simulink model "KTB1_F"  (R2020a)
settings: Solver=ode45  StartTime=0.0  StopTime=120  RelTol=1e-3
libraries: simulink x8
settings Model: Creator=s182032  LastModifiedBy=morebo
settings DataIOCC: ReturnWorkspaceOutputs=off
settings DebuggingCC: MaxConsecutiveZCsMsg=none  ArithmeticOperatorsInVariantConditions=warning
settings SFSimCC: SimUseLocalCustomCode=off  CustomCodeUndefinedFunction=UseInterfaceOnly
settings RTWCC: RTWUseLocalCustomCode=off

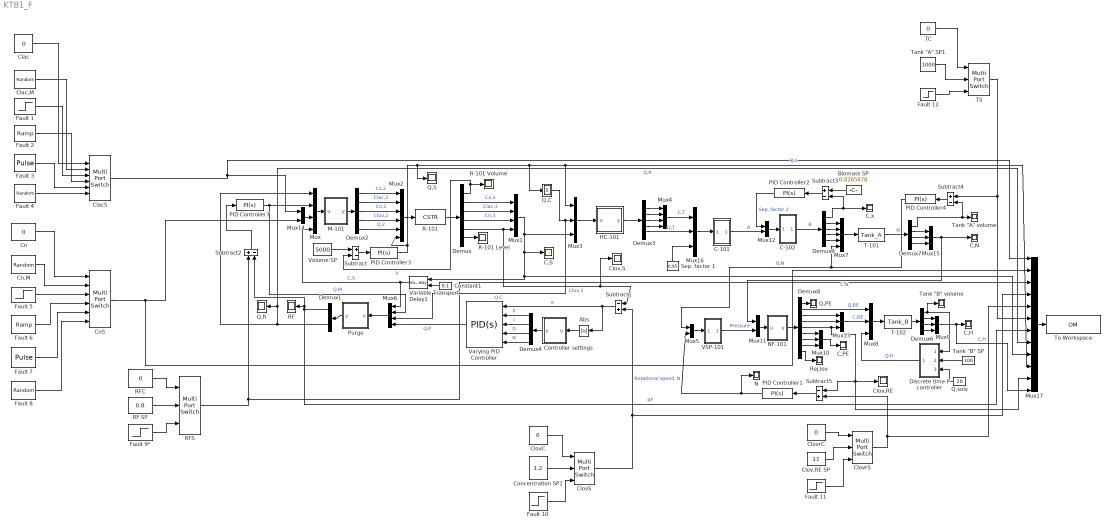
== system KTB1_F ==
  Abs : Abs
  Biomass SP : Constant  Value=0.0265878
  C,H : Scope
  C,N : Scope
  C,PE : Scope
  C,S : Scope
  C,x : Scope
  C-101 : MATLAB Function  TreatAsAtomicUnit=on
  C-102 : MATLAB Function  TreatAsAtomicUnit=on
  Clac : Constant  Value=0
  Clac,M : RandomNumber  Mean=20  Variance=0.001  SampleTime=0.1
  "ClacS " : MultiPortSwitch  DataPortOrder=Zero-based contiguous  Inputs=5  zeroidx=on
  Clov,RE : Scope
  Clov,RE SP : Constant  Value=11
  Clov,S : Scope
  ClovC : Constant  Value=0
  ClovS : MultiPortSwitch  DataPortOrder=Zero-based contiguous  Inputs=2  zeroidx=on
  ClovrC : Constant  Value=0
  "ClovrS " : MultiPortSwitch  DataPortOrder=Zero-based contiguous  Inputs=2  zeroidx=on
  Cn : Constant  Value=0
  Cn,M : RandomNumber  Mean=4  Variance=0.001  SampleTime=0.1
  CnS : MultiPortSwitch  DataPortOrder=Zero-based contiguous  Inputs=5  zeroidx=on
  Concentration SP1 : Constant  Value=1.2
  Constant1 : Constant  Value=0.1
  Controller settings : MATLAB Function  TreatAsAtomicUnit=on
  Demux : Demux  Outputs=6
  Demux1 : Demux  Outputs=2
  Demux2 : Demux  Outputs=5
  Demux3 : Demux  Outputs=5
  Demux4 : Demux
  Demux6 : Demux
  Demux7 : Demux
  Demux8 : Demux  Outputs=9
  Demux9 : Demux  Outputs=5
  Discrete time P controller : Subsystem
  Fault 1 : Step  Time=10  Before=20  After=16  SampleTime=0
  Fault 10 : Step  Time=10.3  Before=1.2  After=1.18  SampleTime=0
  Fault 11 : Step  Before=10.4  After=9  SampleTime=0
  Fault 12 : Step  Time=10.4  Before=1000  After=1050  SampleTime=0
  Fault 2 : simulink/Sources/Ramp  slope=-0.2  start=10  InitialOutput=20
  Fault 3 : DiscretePulseGenerator  Amplitude=20  Period=30  PulseWidth=10  SampleTime=2
  Fault 4 : RandomNumber  Mean=20  Variance=4  SampleTime=0.1
  Fault 5 : Step  Time=10.1  Before=4  After=4.8  SampleTime=0
  Fault 6 : simulink/Sources/Ramp  slope=0.05  start=10  InitialOutput=4
  Fault 7 : DiscretePulseGenerator  Amplitude=4  Period=30  PulseWidth=10  SampleTime=2
  Fault 8 : RandomNumber  Mean=4  Variance=3  SampleTime=0.1
  Fault 9* : Step  Time=10.2  Before=0.8  After=0.84  SampleTime=0
  HC-101 : MATLAB Function  TreatAsAtomicUnit=on
  M-101 : MATLAB Function  TreatAsAtomicUnit=on
  Mux{,1,4,6} (4 alike) : Mux
  Mux{3,8..10,13,15..16} (7 alike) : Mux  Inputs=3
  Mux{5,11..12,14} (4 alike) : Mux  Inputs=2
  Mux17 : Mux  Inputs=12
  Mux2 : Mux  Inputs=6
  Mux7 : Mux  Inputs=5
  N : Scope
  NF-101 : MATLAB Function  TreatAsAtomicUnit=on
  PID Controller1 : simulink/Continuous/PID Controller  Controller=PI  Form=Parallel  TimeDomain=Continuous-time  UseExternalTs=off  SampleTime=-1  IntegratorMethod=Forward Euler  FilterMethod=Forward Euler  ControllerParametersSource=internal  P=0.234567821807165  I=0.999999996666666*0.234567821807165  D=0  UseFilter=on  N=100  TunerSelectOption=Transfer Function Based (PID Tuner App)  InitialConditionSource=internal  InitialConditionForIntegrator=3000  InitialConditionForFilter=0  DifferentiatorICPrevScaledInput=0  ExternalReset=none  TrackingMode=off  Kt=1  LimitOutput=on  UpperSaturationLimit=inf  LowerSaturationLimit=0  LinearizeAsGain=on  AntiWindupMode=clamping  Kb=1  POutMin=[]  POutMax=[]  IOutMin=[]  IOutMax=[]  DOutMin=[]  DOutMax=[]  NOutMin=[]  NOutMax=[]  SumOutMin=[]  SumOutMax=[]  SaturationOutMin=[]  SaturationOutMax=[]  PParamMin=[]  PParamMax=[]  IParamMin=[]  IParamMax=[]  DParamMin=[]  DParamMax=[]  NParamMin=[]  NParamMax=[]  KbParamMin=[]  KbParamMax=[]  KtParamMin=[]  KtParamMax=[]  KbOutMin=[]  KbOutMax=[]  KtOutMin=[]  KtOutMax=[]  IntegratorOutMin=[]  IntegratorOutMax=[]  FilterOutMin=[]  FilterOutMax=[]  SumI1OutMin=[]  SumI1OutMax=[]  SumI2OutMin=[]  SumI2OutMax=[]  SumI3OutMin=[]  SumI3OutMax=[]  SumI4OutMin=[]  SumI4OutMax=[]  SumDOutMin=[]  SumDOutMax=[]  DifferentiatorOutMin=[]  DifferentiatorOutMax=[]  FilterDiffOutCoefMin=[]  FilterDiffOutCoefMax=[]  ReciprocalOutMin=[]  ReciprocalOutMax=[]  SumDenOutMin=[]  SumDenOutMax=[]  SumNumOutMin=[]  SumNumOutMax=[]  DivideOutMin=[]  DivideOutMax=[]  UdiffTsProdOutMin=[]  UdiffTsProdOutMax=[]  NTsProdOutMin=[]  NTsProdOutMax=[]  UintegralTsProdOutMin=[]  UintegralTsProdOutMax=[]  UngainTsProdOutMin=[]  UngainTsProdOutMax=[]  IntegratorContinuousStateAttributes=''  IntegratorStateMustResolveToSignalObject=off  IntegratorRTWStateStorageClass=Auto  FilterContinuousStateAttributes=''  FilterStateMustResolveToSignalObject=off  FilterRTWStateStorageClass=Auto  ParallelPVariant=InternalParameters  IdealPVariant=Disabled  IVariant=InternalParameters  DVariant=Disabled  IntegratorVariant=Continuous  SatVariant=Enabled  AWVariant=ContClampingParallel  PCopyVariant=Disabled  TRVariant=Disabled  FdbkBlocksVariant=Forward  IdealPFdbkVariant=Disabled  SatFdbkVariant=Disabled  DerivativeFilterVariant=Disabled  NVariant=Disabled  NCopyVariant=Disabled_SignalSpec  FilterICVariant=Disabled  IntegratorICVariant=InternalICs  ExternalResetVariant=Disabled  TRSumVariant=Passthrough  SumFdbkVariant=Disabled  SumVariant=Sum_PI  TsampFilterVariant=InternalTs  TsampNgainVariant=Passthrough  TsampIntegralVariant=Passthrough
  PID Controller2 : simulink/Continuous/PID Controller  Controller=PI  Form=Parallel  TimeDomain=Continuous-time  UseExternalTs=off  SampleTime=-1  IntegratorMethod=Forward Euler  FilterMethod=Forward Euler  ControllerParametersSource=internal  P=-0.000476190628986061  I=9.99999996666667*(-0.000476190628986061)  D=0  UseFilter=on  N=100  TunerSelectOption=Transfer Function Based (PID Tuner App)  InitialConditionSource=internal  InitialConditionForIntegrator=0.95  InitialConditionForFilter=0  DifferentiatorICPrevScaledInput=0  ExternalReset=none  TrackingMode=off  Kt=1  LimitOutput=on  UpperSaturationLimit=0.98  LowerSaturationLimit=0  LinearizeAsGain=on  AntiWindupMode=clamping  Kb=1  POutMin=[]  POutMax=[]  IOutMin=[]  IOutMax=[]  DOutMin=[]  DOutMax=[]  NOutMin=[]  NOutMax=[]  SumOutMin=[]  SumOutMax=[]  SaturationOutMin=[]  SaturationOutMax=[]  PParamMin=[]  PParamMax=[]  IParamMin=[]  IParamMax=[]  DParamMin=[]  DParamMax=[]  NParamMin=[]  NParamMax=[]  KbParamMin=[]  KbParamMax=[]  KtParamMin=[]  KtParamMax=[]  KbOutMin=[]  KbOutMax=[]  KtOutMin=[]  KtOutMax=[]  IntegratorOutMin=[]  IntegratorOutMax=[]  FilterOutMin=[]  FilterOutMax=[]  SumI1OutMin=[]  SumI1OutMax=[]  SumI2OutMin=[]  SumI2OutMax=[]  SumI3OutMin=[]  SumI3OutMax=[]  SumI4OutMin=[]  SumI4OutMax=[]  SumDOutMin=[]  SumDOutMax=[]  DifferentiatorOutMin=[]  DifferentiatorOutMax=[]  FilterDiffOutCoefMin=[]  FilterDiffOutCoefMax=[]  ReciprocalOutMin=[]  ReciprocalOutMax=[]  SumDenOutMin=[]  SumDenOutMax=[]  SumNumOutMin=[]  SumNumOutMax=[]  DivideOutMin=[]  DivideOutMax=[]  UdiffTsProdOutMin=[]  UdiffTsProdOutMax=[]  NTsProdOutMin=[]  NTsProdOutMax=[]  UintegralTsProdOutMin=[]  UintegralTsProdOutMax=[]  UngainTsProdOutMin=[]  UngainTsProdOutMax=[]  IntegratorContinuousStateAttributes=''  IntegratorStateMustResolveToSignalObject=off  IntegratorRTWStateStorageClass=Auto  FilterContinuousStateAttributes=''  FilterStateMustResolveToSignalObject=off  FilterRTWStateStorageClass=Auto  ParallelPVariant=InternalParameters  IdealPVariant=Disabled  IVariant=InternalParameters  DVariant=Disabled  IntegratorVariant=Continuous  SatVariant=Enabled  AWVariant=ContClampingParallel  PCopyVariant=Disabled  TRVariant=Disabled  FdbkBlocksVariant=Forward  IdealPFdbkVariant=Disabled  SatFdbkVariant=Disabled  DerivativeFilterVariant=Disabled  NVariant=Disabled  NCopyVariant=Disabled_SignalSpec  FilterICVariant=Disabled  IntegratorICVariant=InternalICs  ExternalResetVariant=Disabled  TRSumVariant=Passthrough  SumFdbkVariant=Disabled  SumVariant=Sum_PI  TsampFilterVariant=InternalTs  TsampNgainVariant=Passthrough  TsampIntegralVariant=Passthrough
  PID Controller3 : simulink/Continuous/PID Controller  Controller=PI  Form=Parallel  TimeDomain=Continuous-time  UseExternalTs=off  SampleTime=-1  IntegratorMethod=Forward Euler  FilterMethod=Forward Euler  ControllerParametersSource=internal  P=-1/0.4/0.2  I=-1/0.4/0.2/4/0.2  D=0  UseFilter=on  N=100  TunerSelectOption=Transfer Function Based (PID Tuner App)  InitialConditionSource=internal  InitialConditionForIntegrator=64.0830509473650  InitialConditionForFilter=0  DifferentiatorICPrevScaledInput=0  ExternalReset=none  TrackingMode=off  Kt=1  LimitOutput=on  UpperSaturationLimit=inf  LowerSaturationLimit=0  LinearizeAsGain=on  AntiWindupMode=clamping  Kb=1  POutMin=[]  POutMax=[]  IOutMin=[]  IOutMax=[]  DOutMin=[]  DOutMax=[]  NOutMin=[]  NOutMax=[]  SumOutMin=[]  SumOutMax=[]  SaturationOutMin=[]  SaturationOutMax=[]  PParamMin=[]  PParamMax=[]  IParamMin=[]  IParamMax=[]  DParamMin=[]  DParamMax=[]  NParamMin=[]  NParamMax=[]  KbParamMin=[]  KbParamMax=[]  KtParamMin=[]  KtParamMax=[]  KbOutMin=[]  KbOutMax=[]  KtOutMin=[]  KtOutMax=[]  IntegratorOutMin=[]  IntegratorOutMax=[]  FilterOutMin=[]  FilterOutMax=[]  SumI1OutMin=[]  SumI1OutMax=[]  SumI2OutMin=[]  SumI2OutMax=[]  SumI3OutMin=[]  SumI3OutMax=[]  SumI4OutMin=[]  SumI4OutMax=[]  SumDOutMin=[]  SumDOutMax=[]  DifferentiatorOutMin=[]  DifferentiatorOutMax=[]  FilterDiffOutCoefMin=[]  FilterDiffOutCoefMax=[]  ReciprocalOutMin=[]  ReciprocalOutMax=[]  SumDenOutMin=[]  SumDenOutMax=[]  SumNumOutMin=[]  SumNumOutMax=[]  DivideOutMin=[]  DivideOutMax=[]  UdiffTsProdOutMin=[]  UdiffTsProdOutMax=[]  NTsProdOutMin=[]  NTsProdOutMax=[]  UintegralTsProdOutMin=[]  UintegralTsProdOutMax=[]  UngainTsProdOutMin=[]  UngainTsProdOutMax=[]  IntegratorContinuousStateAttributes=''  IntegratorStateMustResolveToSignalObject=off  IntegratorRTWStateStorageClass=Auto  FilterContinuousStateAttributes=''  FilterStateMustResolveToSignalObject=off  FilterRTWStateStorageClass=Auto  ParallelPVariant=InternalParameters  IdealPVariant=Disabled  IVariant=InternalParameters  DVariant=Disabled  IntegratorVariant=Continuous  SatVariant=Enabled  AWVariant=ContClampingParallel  PCopyVariant=Disabled  TRVariant=Disabled  FdbkBlocksVariant=Forward  IdealPFdbkVariant=Disabled  SatFdbkVariant=Disabled  DerivativeFilterVariant=Disabled  NVariant=Disabled  NCopyVariant=Disabled_SignalSpec  FilterICVariant=Disabled  IntegratorICVariant=InternalICs  ExternalResetVariant=Disabled  TRSumVariant=Passthrough  SumFdbkVariant=Disabled  SumVariant=Sum_PI  TsampFilterVariant=InternalTs  TsampNgainVariant=Passthrough  TsampIntegralVariant=Passthrough
  PID Controller4 : simulink/Continuous/PID Controller  Controller=PI  Form=Parallel  TimeDomain=Continuous-time  UseExternalTs=off  SampleTime=-1  IntegratorMethod=Forward Euler  FilterMethod=Forward Euler  ControllerParametersSource=internal  P=-1/140  I=-1/4/140/140  D=0  UseFilter=on  N=100  TunerSelectOption=Transfer Function Based (PID Tuner App)  InitialConditionSource=internal  InitialConditionForIntegrator=25.6332203789471  InitialConditionForFilter=0  DifferentiatorICPrevScaledInput=0  ExternalReset=none  TrackingMode=off  Kt=1  LimitOutput=on  UpperSaturationLimit=inf  LowerSaturationLimit=0  LinearizeAsGain=on  AntiWindupMode=clamping  Kb=1  POutMin=[]  POutMax=[]  IOutMin=[]  IOutMax=[]  DOutMin=[]  DOutMax=[]  NOutMin=[]  NOutMax=[]  SumOutMin=[]  SumOutMax=[]  SaturationOutMin=[]  SaturationOutMax=[]  PParamMin=[]  PParamMax=[]  IParamMin=[]  IParamMax=[]  DParamMin=[]  DParamMax=[]  NParamMin=[]  NParamMax=[]  KbParamMin=[]  KbParamMax=[]  KtParamMin=[]  KtParamMax=[]  KbOutMin=[]  KbOutMax=[]  KtOutMin=[]  KtOutMax=[]  IntegratorOutMin=[]  IntegratorOutMax=[]  FilterOutMin=[]  FilterOutMax=[]  SumI1OutMin=[]  SumI1OutMax=[]  SumI2OutMin=[]  SumI2OutMax=[]  SumI3OutMin=[]  SumI3OutMax=[]  SumI4OutMin=[]  SumI4OutMax=[]  SumDOutMin=[]  SumDOutMax=[]  DifferentiatorOutMin=[]  DifferentiatorOutMax=[]  FilterDiffOutCoefMin=[]  FilterDiffOutCoefMax=[]  ReciprocalOutMin=[]  ReciprocalOutMax=[]  SumDenOutMin=[]  SumDenOutMax=[]  SumNumOutMin=[]  SumNumOutMax=[]  DivideOutMin=[]  DivideOutMax=[]  UdiffTsProdOutMin=[]  UdiffTsProdOutMax=[]  NTsProdOutMin=[]  NTsProdOutMax=[]  UintegralTsProdOutMin=[]  UintegralTsProdOutMax=[]  UngainTsProdOutMin=[]  UngainTsProdOutMax=[]  IntegratorContinuousStateAttributes=''  IntegratorStateMustResolveToSignalObject=off  IntegratorRTWStateStorageClass=Auto  FilterContinuousStateAttributes=''  FilterStateMustResolveToSignalObject=off  FilterRTWStateStorageClass=Auto  ParallelPVariant=InternalParameters  IdealPVariant=Disabled  IVariant=InternalParameters  DVariant=Disabled  IntegratorVariant=Continuous  SatVariant=Enabled  AWVariant=ContClampingParallel  PCopyVariant=Disabled  TRVariant=Disabled  FdbkBlocksVariant=Forward  IdealPFdbkVariant=Disabled  SatFdbkVariant=Disabled  DerivativeFilterVariant=Disabled  NVariant=Disabled  NCopyVariant=Disabled_SignalSpec  FilterICVariant=Disabled  IntegratorICVariant=InternalICs  ExternalResetVariant=Disabled  TRSumVariant=Passthrough  SumFdbkVariant=Disabled  SumVariant=Sum_PI  TsampFilterVariant=InternalTs  TsampNgainVariant=Passthrough  TsampIntegralVariant=Passthrough
  PID Controller7 : simulink/Continuous/PID Controller  Controller=PI  Form=Parallel  TimeDomain=Continuous-time  UseExternalTs=off  SampleTime=-1  IntegratorMethod=Forward Euler  FilterMethod=Forward Euler  ControllerParametersSource=internal  P=4.68116891262785/100  I=30.3539293345611/100  D=0  UseFilter=on  N=100  TunerSelectOption=Transfer Function Based (PID Tuner App)  InitialConditionSource=internal  InitialConditionForIntegrator=35.6016949707568  InitialConditionForFilter=0  DifferentiatorICPrevScaledInput=0  ExternalReset=none  TrackingMode=off  Kt=1  LimitOutput=on  UpperSaturationLimit=inf  LowerSaturationLimit=0  LinearizeAsGain=on  AntiWindupMode=clamping  Kb=1  POutMin=[]  POutMax=[]  IOutMin=[]  IOutMax=[]  DOutMin=[]  DOutMax=[]  NOutMin=[]  NOutMax=[]  SumOutMin=[]  SumOutMax=[]  SaturationOutMin=[]  SaturationOutMax=[]  PParamMin=[]  PParamMax=[]  IParamMin=[]  IParamMax=[]  DParamMin=[]  DParamMax=[]  NParamMin=[]  NParamMax=[]  KbParamMin=[]  KbParamMax=[]  KtParamMin=[]  KtParamMax=[]  KbOutMin=[]  KbOutMax=[]  KtOutMin=[]  KtOutMax=[]  IntegratorOutMin=[]  IntegratorOutMax=[]  FilterOutMin=[]  FilterOutMax=[]  SumI1OutMin=[]  SumI1OutMax=[]  SumI2OutMin=[]  SumI2OutMax=[]  SumI3OutMin=[]  SumI3OutMax=[]  SumI4OutMin=[]  SumI4OutMax=[]  SumDOutMin=[]  SumDOutMax=[]  DifferentiatorOutMin=[]  DifferentiatorOutMax=[]  FilterDiffOutCoefMin=[]  FilterDiffOutCoefMax=[]  ReciprocalOutMin=[]  ReciprocalOutMax=[]  SumDenOutMin=[]  SumDenOutMax=[]  SumNumOutMin=[]  SumNumOutMax=[]  DivideOutMin=[]  DivideOutMax=[]  UdiffTsProdOutMin=[]  UdiffTsProdOutMax=[]  NTsProdOutMin=[]  NTsProdOutMax=[]  UintegralTsProdOutMin=[]  UintegralTsProdOutMax=[]  UngainTsProdOutMin=[]  UngainTsProdOutMax=[]  IntegratorContinuousStateAttributes=''  IntegratorStateMustResolveToSignalObject=off  IntegratorRTWStateStorageClass=Auto  FilterContinuousStateAttributes=''  FilterStateMustResolveToSignalObject=off  FilterRTWStateStorageClass=Auto  ParallelPVariant=InternalParameters  IdealPVariant=Disabled  IVariant=InternalParameters  DVariant=Disabled  IntegratorVariant=Continuous  SatVariant=Enabled  AWVariant=ContClampingParallel  PCopyVariant=Disabled  TRVariant=Disabled  FdbkBlocksVariant=Forward  IdealPFdbkVariant=Disabled  SatFdbkVariant=Disabled  DerivativeFilterVariant=Disabled  NVariant=Disabled  NCopyVariant=Disabled_SignalSpec  FilterICVariant=Disabled  IntegratorICVariant=InternalICs  ExternalResetVariant=Disabled  TRSumVariant=Passthrough  SumFdbkVariant=Disabled  SumVariant=Sum_PI  TsampFilterVariant=InternalTs  TsampNgainVariant=Passthrough  TsampIntegralVariant=Passthrough
  Purge : MATLAB Function  TreatAsAtomicUnit=on
  Q,C : Subsystem
  Q,PE : Scope
  Q,R : Scope
  Q,S : Scope
  Q,solv : Constant  Value=20
  R-101 : S-Function  FunctionName=CSTR  SFunctionDeploymentMode=off  EnableBusSupport=off
  R-101 Level : Scope
  R-101 Volume : Scope
  RF : Scope
  RF SP : Constant  Value=0.8
  RFC : Constant  Value=0
  RFS : MultiPortSwitch  DataPortOrder=Zero-based contiguous  Inputs=2  zeroidx=on
  Rej,lov : Scope
  Sep. factor 1 : Constant  Value=0.95
  Subtract{,2..4} (4 alike) : Sum  Inputs=+-
  Subtract1 : Sum  Inputs=-+
  Subtract5 : Sum  Inputs=-+
  T-101 : S-Function  FunctionName=Tank_A  SFunctionDeploymentMode=off  EnableBusSupport=off
  T-102 : S-Function  FunctionName=Tank_B  SFunctionDeploymentMode=off  EnableBusSupport=off
  TC : Constant  Value=0
  "TS " : MultiPortSwitch  DataPortOrder=Zero-based contiguous  Inputs=2  zeroidx=on
  "Tank \"A\" SP1" : Constant  Value=1000
  "Tank \"A\" volume" : Scope
  "Tank \"B\" SP" : Constant  Value=100
  "Tank \"B\" volume" : Scope
  To Workspace : ToWorkspace  VariableName=OM  SaveFormat=Timeseries  SampleTime=-1
  VSP-101 : MATLAB Function  TreatAsAtomicUnit=on
  Variable Transport Delay1 : VariableTransportDelay  VariableDelayType=Variable transport delay  MaximumDelay=10  InitialOutput=[106.351163614666 14.8096563646109 2.51553709810012 1.20000000000003]  MaximumPoints=80000
  Varying PID Controller : simulink/Continuous/PID Controller  Controller=PID  Form=Parallel  TimeDomain=Continuous-time  UseExternalTs=off  SampleTime=-1  IntegratorMethod=Forward Euler  FilterMethod=Forward Euler  ControllerParametersSource=external  P=1  I=1  D=0  UseFilter=on  N=100  TunerSelectOption=Transfer Function Based (PID Tuner App)  InitialConditionSource=internal  InitialConditionForIntegrator=9.96847459181301  InitialConditionForFilter=0  DifferentiatorICPrevScaledInput=0  ExternalReset=none  TrackingMode=off  Kt=1  LimitOutput=on  UpperSaturationLimit=inf  LowerSaturationLimit=0  LinearizeAsGain=on  AntiWindupMode=none  Kb=1  POutMin=[]  POutMax=[]  IOutMin=[]  IOutMax=[]  DOutMin=[]  DOutMax=[]  NOutMin=[]  NOutMax=[]  SumOutMin=[]  SumOutMax=[]  SaturationOutMin=[]  SaturationOutMax=[]  PParamMin=[]  PParamMax=[]  IParamMin=[]  IParamMax=[]  DParamMin=[]  DParamMax=[]  NParamMin=[]  NParamMax=[]  KbParamMin=[]  KbParamMax=[]  KtParamMin=[]  KtParamMax=[]  KbOutMin=[]  KbOutMax=[]  KtOutMin=[]  KtOutMax=[]  IntegratorOutMin=[]  IntegratorOutMax=[]  FilterOutMin=[]  FilterOutMax=[]  SumI1OutMin=[]  SumI1OutMax=[]  SumI2OutMin=[]  SumI2OutMax=[]  SumI3OutMin=[]  SumI3OutMax=[]  SumI4OutMin=[]  SumI4OutMax=[]  SumDOutMin=[]  SumDOutMax=[]  DifferentiatorOutMin=[]  DifferentiatorOutMax=[]  FilterDiffOutCoefMin=[]  FilterDiffOutCoefMax=[]  ReciprocalOutMin=[]  ReciprocalOutMax=[]  SumDenOutMin=[]  SumDenOutMax=[]  SumNumOutMin=[]  SumNumOutMax=[]  DivideOutMin=[]  DivideOutMax=[]  UdiffTsProdOutMin=[]  UdiffTsProdOutMax=[]  NTsProdOutMin=[]  NTsProdOutMax=[]  UintegralTsProdOutMin=[]  UintegralTsProdOutMax=[]  UngainTsProdOutMin=[]  UngainTsProdOutMax=[]  IntegratorContinuousStateAttributes=''  IntegratorStateMustResolveToSignalObject=off  IntegratorRTWStateStorageClass=Auto  FilterContinuousStateAttributes=''  FilterStateMustResolveToSignalObject=off  FilterRTWStateStorageClass=Auto  ParallelPVariant=ExternalParameters  IdealPVariant=Disabled  IVariant=ExternalParameters  DVariant=ExternalParameters  IntegratorVariant=Continuous  SatVariant=Enabled  AWVariant=Passthrough  PCopyVariant=Disabled  TRVariant=Disabled  FdbkBlocksVariant=Forward  IdealPFdbkVariant=Disabled  SatFdbkVariant=Disabled  DerivativeFilterVariant=ContFilter  NVariant=ExternalParameters  NCopyVariant=Disabled  FilterICVariant=InternalICsFilter  IntegratorICVariant=InternalICs  ExternalResetVariant=Disabled  TRSumVariant=Passthrough  SumFdbkVariant=Disabled  SumVariant=Sum_PID  TsampFilterVariant=InternalTs  TsampNgainVariant=Passthrough  TsampIntegralVariant=Passthrough
  Volume SP : Constant  Value=5000
  wires:
  Demux4/1 -> Varying PID Controller/2  "P"
  Subtract1/1 -> Abs/1, Varying PID Controller/1  "e"
  Demux4/2 -> Varying PID Controller/3  "I"
  PID Controller7/1 -> Mux6/2, Mux/2  "Q,M"
  Varying PID Controller/1 -> Mux6/4  "Q,P"
  Demux2/5 -> Mux2/5  "Q,2"
  Mux6/1 -> Purge/1(u)
  Demux2/4 -> Mux2/4  "Clov,2"
  Demux3/1 -> Mux4/1
  Purge/1(y) -> Demux1/1
  Demux2/3 -> Mux2/3  "Cn,2"
  Demux3/2 -> Mux4/2
  Demux3/3 -> Mux4/3
  HC-101/1(y) -> Demux3/1
  Mux3/1 -> HC-101/1(u)
  Demux2/2 -> Mux2/2  "Clac,2"
  PID Controller3/1 -> Mux2/6, Q,S/1, Mux17/10, Mux3/1, Q,C/1(Qs)  "Q,S"
  Demux/1 -> R-101 Volume/1, Subtract/2  "V"
  Demux/2 -> Mux1/1  "Cx,3"
  Demux/3 -> Mux1/2  "Clac,3"
  Mux/1 -> M-101/1(u)
  Mux2/1 -> R-101/1
  Demux2/1 -> Mux2/1  "Cx,2"
  Variable Transport Delay1/1 -> Mux/4, Mux6/1  "C,S"
  R-101/1 -> Demux/1
  Mux1/1 -> C,S/1, Variable Transport Delay1/1, Mux17/9, Mux3/3
  Constant1/1 -> Variable Transport Delay1/2
  M-101/1(y) -> Demux2/1
  Demux/4 -> Mux1/3  "Cn,3"
  Demux/5 -> Clov,S/1, Subtract1/1, Mux1/4  "Clov,3"
  Subtract/1 -> PID Controller3/1
  Demux3/4 -> Mux4/4
  Cn,M/1 -> CnS/2
  Demux/6 -> R-101 Level/1
  Mux14/1 -> Mux/3
  Demux1/2 -> Mux17/8, Q,R/1, Mux/1  "Q,R"
  Volume SP/1 -> Subtract/1
  Demux1/1 -> Mux17/7, RF/1, Subtract2/2  "RF"
  Abs/1 -> Controller settings/1(u)
  Controller settings/1(y) -> Demux4/1
  Demux4/3 -> Varying PID Controller/4  "D"
  Demux4/4 -> Varying PID Controller/5  "N"
  Subtract2/1 -> PID Controller7/1
  Q,C/1(Qc) -> Mux6/3, Mux3/2  "Q,C"
  Demux6/1 -> Discrete time P controller/1(In1), "Tank \"B\" volume"/1
  Discrete time P controller/1(Q,H) -> Mux8/3  "Q,H"
  Q,solv/1 -> Discrete time P controller/3(In3)
  "Tank \"B\" SP"/1 -> Discrete time P controller/2(In2)
  Demux9/4 -> Mux7/3
  Subtract3/1 -> PID Controller2/1
  C-102/1(y) -> Demux9/1  "B"
  Demux8/9 -> Rej,lov/1
  PID Controller1/1 -> Mux5/2, N/1  "Rotational speed, N"
  Demux9/1 -> C,x/1, Subtract3/2
  Demux7/3 -> Mux15/2
  Demux8/8 -> Mux10/3
  Demux9/2 -> Mux7/1
  Mux5/1 -> VSP-101/1(u)
  VSP-101/1(y) -> Mux11/2  "Pressure"
  Demux6/2 -> Mux9/1
  T-102/1 -> Demux6/1
  Demux9/5 -> Mux7/4
  Demux8/2 -> Mux8/1  "Q,RE"
  Demux6/3 -> Mux9/2
  Mux15/1 -> C,N/1, Mux11/1  "C,N"
  Mux7/1 -> T-101/1
  Demux9/3 -> Mux7/2
  Demux8/3 -> Mux13/1
  Demux8/5 -> Mux17/11, Subtract5/1, Clov,RE/1, Mux13/3
  Mux8/1 -> T-102/1
  Mux10/1 -> C,PE/1
  Demux8/4 -> Mux13/2
  Subtract4/1 -> PID Controller4/1
  PID Controller4/1 -> Mux5/1, Mux7/5  "Q,N"
  Subtract5/1 -> PID Controller1/1
  Demux8/7 -> Mux10/2
  Demux6/4 -> Mux9/3
  Demux7/1 -> "Tank \"A\" volume"/1, Subtract4/2
  Mux16/1 -> C-101/1(u)
  Sep. factor 1/1 -> Mux16/3
  Mux11/1 -> NF-101/1(u)
  NF-101/1(y) -> Demux8/1
  Mux9/1 -> Mux17/12, C,H/1  "C,H"
  T-101/1 -> Demux7/1  "N"
  Mux13/1 -> Mux8/2  "C,RE"
  Mux12/1 -> C-102/1(u)
  Biomass SP/1 -> Subtract3/1
  Demux8/6 -> Mux10/1
  Demux7/4 -> Mux15/3
  Demux8/1 -> Q,PE/1
  C-101/1(y) -> Mux12/2  "A"
  Demux7/2 -> Mux15/1
  PID Controller2/1 -> Mux12/1  "Sep. factor 2"
  Mux4/1 -> Mux16/1  "C,T"
  Demux3/5 -> Mux16/2  "Q,T"
  Mux17/1 -> To Workspace/1
  Fault 1/1 -> "ClacS "/3
  Fault 2/1 -> "ClacS "/4
  "ClacS "/1 -> Mux17/1, Mux14/1
  Clac,M/1 -> "ClacS "/2
  Fault 3/1 -> "ClacS "/5
  Fault 4/1 -> "ClacS "/6
  CnS/1 -> Mux17/2, Mux14/2
  Fault 5/1 -> CnS/3
  Fault 6/1 -> CnS/4
  Fault 7/1 -> CnS/5
  Clac/1 -> "ClacS "/1
  Cn/1 -> CnS/1
  Fault 8/1 -> CnS/6
  RFC/1 -> RFS/1
  RF SP/1 -> RFS/2
  Fault 9*/1 -> RFS/3
  RFS/1 -> Subtract2/1, Mux17/3
  ClovrC/1 -> "ClovrS "/1
  "ClovrS "/1 -> Mux17/5, Subtract5/2
  Clov,RE SP/1 -> "ClovrS "/2
  Fault 11/1 -> "ClovrS "/3
  "Tank \"A\" SP1"/1 -> "TS "/2
  TC/1 -> "TS "/1
  Fault 12/1 -> "TS "/3
  "TS "/1 -> Mux17/6, Subtract4/1
  Concentration SP1/1 -> ClovS/2
  ClovC/1 -> ClovS/1
  Fault 10/1 -> ClovS/3
  ClovS/1 -> Mux17/4, Subtract1/2

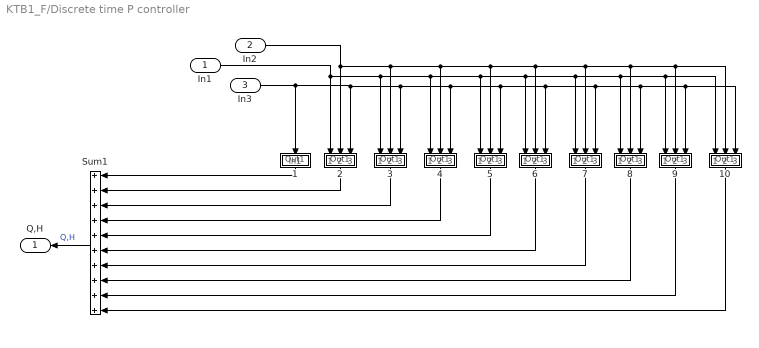
== system KTB1_F/Discrete time P controller ==
  In1 : Inport
  In2 : Inport  Port=2
  In3 : Inport  Port=3
  1 : Subsystem
  10 : Subsystem
  2 : Subsystem
  3 : Subsystem
  4 : Subsystem
  5 : Subsystem
  6 : Subsystem
  7 : Subsystem
  8 : Subsystem
  9 : Subsystem
  Sum1 : Sum  Inputs=++++++++++
  Q,H : Outport  VectorParamsAs1DForOutWhenUnconnected=off
  wires:
  In3/1 -> 3/3(In3), 4/3(In3), 6/3(In3), 7/3(In3), 8/3(In3), 10/3(In3), 9/3(In3), 5/3(In3), 2/3(In3), 1/1(In1)
  In2/1 -> 2/2(In2), 3/2(In2), 4/2(In2), 5/2(In2), 6/2(In2), 8/2(In2), 10/2(In2), 9/2(In2), 7/2(In2)
  7/1(Out1) -> Sum1/7
  3/1(Out1) -> Sum1/3
  4/1(Out1) -> Sum1/4
  2/1(Out1) -> Sum1/2
  6/1(Out1) -> Sum1/6
  8/1(Out1) -> Sum1/8
  10/1(Out1) -> Sum1/10
  9/1(Out1) -> Sum1/9
  5/1(Out1) -> Sum1/5
  Sum1/1 -> Q,H/1  "Q,H"
  1/1(Out1) -> Sum1/1
  In1/1 -> 4/1(In1), 5/1(In1), 6/1(In1), 7/1(In1), 8/1(In1), 10/1(In1), 9/1(In1), 3/1(In1), 2/1(In1)

== system KTB1_F/Q,C ==
  Qs : Inport
  Product1 : Product
  Q,C/Q,S : Constant  Value=0.6
  Qc : Outport  VectorParamsAs1DForOutWhenUnconnected=off
  wires:
  Product1/1 -> Qc/1  "Qc"
  Q,C/Q,S/1 -> Product1/1
  Qs/1 -> Product1/2

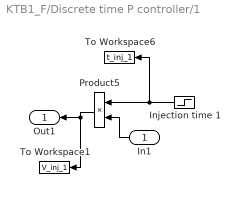
== system KTB1_F/Discrete time P controller/1 ==
  In1 : Inport
  Injection time 1 : Step  Time=(5.1313509526065/20)*6  Before=1  After=0  SampleTime=0
  Product5 : Product
  To Workspace1 : ToWorkspace  VariableName=V_inj_1  SaveFormat=Timeseries  SampleTime=-1
  To Workspace6 : ToWorkspace  VariableName=t_inj_1  SaveFormat=Timeseries  SampleTime=-1
  Out1 : Outport  VectorParamsAs1DForOutWhenUnconnected=off
  wires:
  Product5/1 -> To Workspace1/1, Out1/1
  Injection time 1/1 -> Product5/1, To Workspace6/1
  In1/1 -> Product5/2

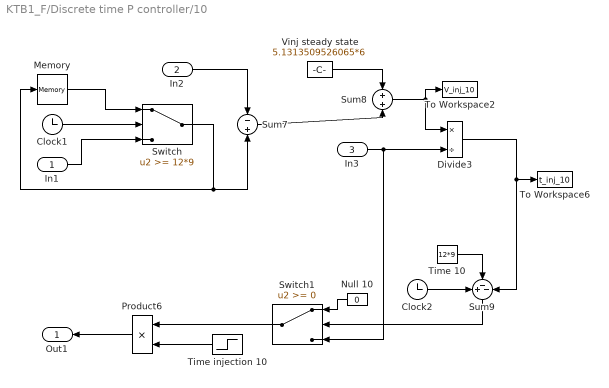
== system KTB1_F/Discrete time P controller/10 ==
  In1 : Inport
  In2 : Inport  Port=2
  In3 : Inport  Port=3
  Clock1 : Clock
  Clock2 : Clock
  Divide3 : Product  Inputs=*/
  Memory : Memory
  Null 10 : Constant  Value=0
  Product6 : Product
  Sum7 : Sum  Inputs=-+
  Sum8 : Sum
  Sum9 : Sum  Inputs=+--
  Switch : Switch  Threshold=12*9
  Switch1 : Switch
  Time 10 : Constant  Value=12*9
  Time injection 10 : Step  Time=12*9  SampleTime=0
  To Workspace2 : ToWorkspace  VariableName=V_inj_10  SaveFormat=Timeseries  SampleTime=-1
  To Workspace6 : ToWorkspace  VariableName=t_inj_10  SaveFormat=Timeseries  SampleTime=-1
  Vinj steady state : Constant  Value=5.1313509526065*6
  Out1 : Outport  VectorParamsAs1DForOutWhenUnconnected=off
  wires:
  In1/1 -> Switch/3
  Time injection 10/1 -> Product6/2
  Switch/1 -> Memory/1, Sum7/2
  Time 10/1 -> Sum9/2
  Switch1/1 -> Product6/1
  Clock1/1 -> Switch/2
  Memory/1 -> Switch/1
  Null 10/1 -> Switch1/1
  Divide3/1 -> Sum9/3, To Workspace6/1
  Clock2/1 -> Sum9/1
  In2/1 -> Sum7/1
  Vinj steady state/1 -> Sum8/1
  In3/1 -> Switch1/3, Divide3/2
  Sum9/1 -> Switch1/2
  Sum7/1 -> Sum8/2
  Product6/1 -> Out1/1
  Sum8/1 -> Divide3/1, To Workspace2/1

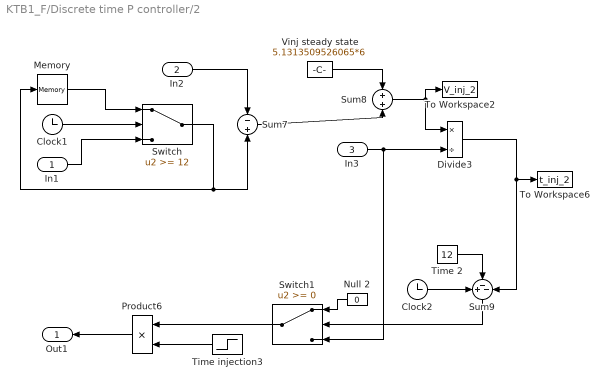
== system KTB1_F/Discrete time P controller/2 ==
  In1 : Inport
  In2 : Inport  Port=2
  In3 : Inport  Port=3
  Clock1 : Clock
  Clock2 : Clock
  Divide3 : Product  Inputs=*/
  Memory : Memory
  Null 2 : Constant  Value=0
  Product6 : Product
  Sum7 : Sum  Inputs=-+
  Sum8 : Sum
  Sum9 : Sum  Inputs=+--
  Switch : Switch  Threshold=12
  Switch1 : Switch
  Time 2 : Constant  Value=12
  Time injection3 : Step  Time=12  SampleTime=0
  To Workspace2 : ToWorkspace  VariableName=V_inj_2  SaveFormat=Timeseries  SampleTime=-1
  To Workspace6 : ToWorkspace  VariableName=t_inj_2  SaveFormat=Timeseries  SampleTime=-1
  Vinj steady state : Constant  Value=5.1313509526065*6
  Out1 : Outport  VectorParamsAs1DForOutWhenUnconnected=off
  wires:
  In1/1 -> Switch/3
  Time injection3/1 -> Product6/2
  Switch/1 -> Memory/1, Sum7/2
  Time 2/1 -> Sum9/2
  Switch1/1 -> Product6/1
  Clock1/1 -> Switch/2
  Memory/1 -> Switch/1
  Null 2/1 -> Switch1/1
  Divide3/1 -> Sum9/3, To Workspace6/1
  Clock2/1 -> Sum9/1
  In2/1 -> Sum7/1
  Vinj steady state/1 -> Sum8/1
  In3/1 -> Switch1/3, Divide3/2
  Sum9/1 -> Switch1/2
  Sum7/1 -> Sum8/2
  Product6/1 -> Out1/1
  Sum8/1 -> Divide3/1, To Workspace2/1

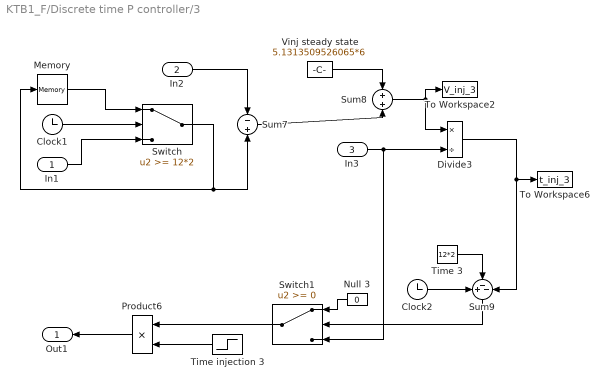
== system KTB1_F/Discrete time P controller/3 ==
  In1 : Inport
  In2 : Inport  Port=2
  In3 : Inport  Port=3
  Clock1 : Clock
  Clock2 : Clock
  Divide3 : Product  Inputs=*/
  Memory : Memory
  Null 3 : Constant  Value=0
  Product6 : Product
  Sum7 : Sum  Inputs=-+
  Sum8 : Sum
  Sum9 : Sum  Inputs=+--
  Switch : Switch  Threshold=12*2
  Switch1 : Switch
  Time 3 : Constant  Value=12*2
  Time injection 3 : Step  Time=12*2  SampleTime=0
  To Workspace2 : ToWorkspace  VariableName=V_inj_3  SaveFormat=Timeseries  SampleTime=-1
  To Workspace6 : ToWorkspace  VariableName=t_inj_3  SaveFormat=Timeseries  SampleTime=-1
  Vinj steady state : Constant  Value=5.1313509526065*6
  Out1 : Outport  VectorParamsAs1DForOutWhenUnconnected=off
  wires:
  In1/1 -> Switch/3
  Time injection 3/1 -> Product6/2
  Switch/1 -> Memory/1, Sum7/2
  Time 3/1 -> Sum9/2
  Switch1/1 -> Product6/1
  Clock1/1 -> Switch/2
  Memory/1 -> Switch/1
  Null 3/1 -> Switch1/1
  Divide3/1 -> Sum9/3, To Workspace6/1
  Clock2/1 -> Sum9/1
  In2/1 -> Sum7/1
  Vinj steady state/1 -> Sum8/1
  In3/1 -> Switch1/3, Divide3/2
  Sum9/1 -> Switch1/2
  Sum7/1 -> Sum8/2
  Product6/1 -> Out1/1
  Sum8/1 -> Divide3/1, To Workspace2/1

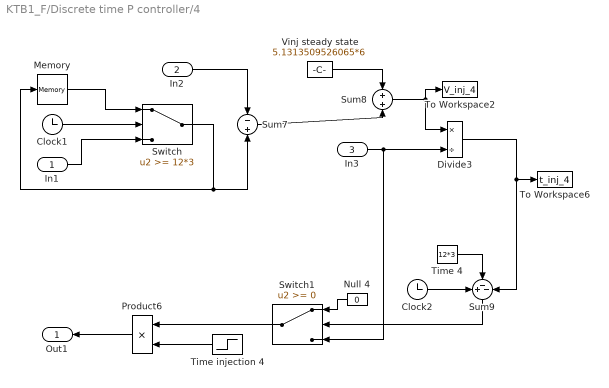
== system KTB1_F/Discrete time P controller/4 ==
  In1 : Inport
  In2 : Inport  Port=2
  In3 : Inport  Port=3
  Clock1 : Clock
  Clock2 : Clock
  Divide3 : Product  Inputs=*/
  Memory : Memory
  Null 4 : Constant  Value=0
  Product6 : Product
  Sum7 : Sum  Inputs=-+
  Sum8 : Sum
  Sum9 : Sum  Inputs=+--
  Switch : Switch  Threshold=12*3
  Switch1 : Switch
  Time 4 : Constant  Value=12*3
  Time injection 4 : Step  Time=12*3  SampleTime=0
  To Workspace2 : ToWorkspace  VariableName=V_inj_4  SaveFormat=Timeseries  SampleTime=-1
  To Workspace6 : ToWorkspace  VariableName=t_inj_4  SaveFormat=Timeseries  SampleTime=-1
  Vinj steady state : Constant  Value=5.1313509526065*6
  Out1 : Outport  VectorParamsAs1DForOutWhenUnconnected=off
  wires:
  In1/1 -> Switch/3
  Time injection 4/1 -> Product6/2
  Switch/1 -> Memory/1, Sum7/2
  Time 4/1 -> Sum9/2
  Switch1/1 -> Product6/1
  Clock1/1 -> Switch/2
  Memory/1 -> Switch/1
  Null 4/1 -> Switch1/1
  Divide3/1 -> Sum9/3, To Workspace6/1
  Clock2/1 -> Sum9/1
  In2/1 -> Sum7/1
  Vinj steady state/1 -> Sum8/1
  In3/1 -> Switch1/3, Divide3/2
  Sum9/1 -> Switch1/2
  Sum7/1 -> Sum8/2
  Product6/1 -> Out1/1
  Sum8/1 -> Divide3/1, To Workspace2/1

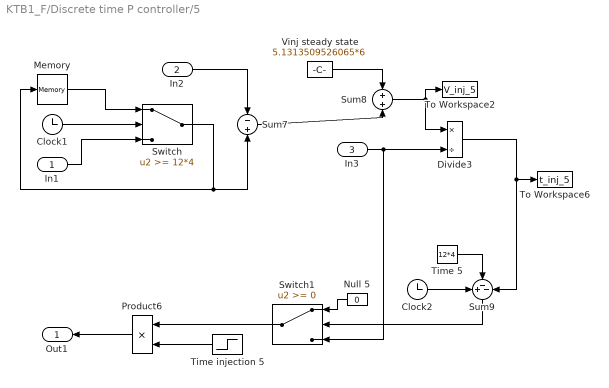
== system KTB1_F/Discrete time P controller/5 ==
  In1 : Inport
  In2 : Inport  Port=2
  In3 : Inport  Port=3
  Clock1 : Clock
  Clock2 : Clock
  Divide3 : Product  Inputs=*/
  Memory : Memory
  Null 5 : Constant  Value=0
  Product6 : Product
  Sum7 : Sum  Inputs=-+
  Sum8 : Sum
  Sum9 : Sum  Inputs=+--
  Switch : Switch  Threshold=12*4
  Switch1 : Switch
  Time 5 : Constant  Value=12*4
  Time injection 5 : Step  Time=12*4  SampleTime=0
  To Workspace2 : ToWorkspace  VariableName=V_inj_5  SaveFormat=Timeseries  SampleTime=-1
  To Workspace6 : ToWorkspace  VariableName=t_inj_5  SaveFormat=Timeseries  SampleTime=-1
  Vinj steady state : Constant  Value=5.1313509526065*6
  Out1 : Outport  VectorParamsAs1DForOutWhenUnconnected=off
  wires:
  In1/1 -> Switch/3
  Time injection 5/1 -> Product6/2
  Switch/1 -> Memory/1, Sum7/2
  Time 5/1 -> Sum9/2
  Switch1/1 -> Product6/1
  Clock1/1 -> Switch/2
  Memory/1 -> Switch/1
  Null 5/1 -> Switch1/1
  Divide3/1 -> Sum9/3, To Workspace6/1
  Clock2/1 -> Sum9/1
  In2/1 -> Sum7/1
  Vinj steady state/1 -> Sum8/1
  In3/1 -> Switch1/3, Divide3/2
  Sum9/1 -> Switch1/2
  Sum7/1 -> Sum8/2
  Product6/1 -> Out1/1
  Sum8/1 -> Divide3/1, To Workspace2/1

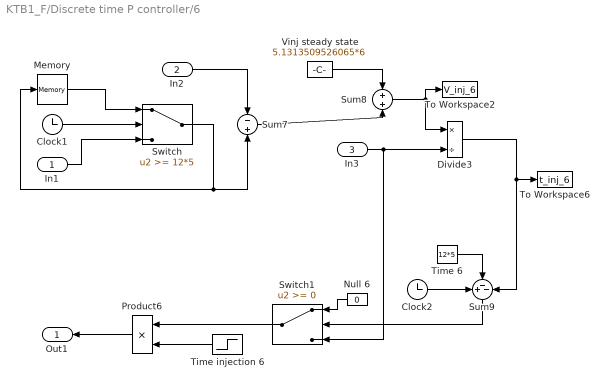
== system KTB1_F/Discrete time P controller/6 ==
  In1 : Inport
  In2 : Inport  Port=2
  In3 : Inport  Port=3
  Clock1 : Clock
  Clock2 : Clock
  Divide3 : Product  Inputs=*/
  Memory : Memory
  Null 6 : Constant  Value=0
  Product6 : Product
  Sum7 : Sum  Inputs=-+
  Sum8 : Sum
  Sum9 : Sum  Inputs=+--
  Switch : Switch  Threshold=12*5
  Switch1 : Switch
  Time 6 : Constant  Value=12*5
  Time injection 6 : Step  Time=12*5  SampleTime=0
  To Workspace2 : ToWorkspace  VariableName=V_inj_6  SaveFormat=Timeseries  SampleTime=-1
  To Workspace6 : ToWorkspace  VariableName=t_inj_6  SaveFormat=Timeseries  SampleTime=-1
  Vinj steady state : Constant  Value=5.1313509526065*6
  Out1 : Outport  VectorParamsAs1DForOutWhenUnconnected=off
  wires:
  In1/1 -> Switch/3
  Time injection 6/1 -> Product6/2
  Switch/1 -> Memory/1, Sum7/2
  Time 6/1 -> Sum9/2
  Switch1/1 -> Product6/1
  Clock1/1 -> Switch/2
  Memory/1 -> Switch/1
  Null 6/1 -> Switch1/1
  Divide3/1 -> Sum9/3, To Workspace6/1
  Clock2/1 -> Sum9/1
  In2/1 -> Sum7/1
  Vinj steady state/1 -> Sum8/1
  In3/1 -> Switch1/3, Divide3/2
  Sum9/1 -> Switch1/2
  Sum7/1 -> Sum8/2
  Product6/1 -> Out1/1
  Sum8/1 -> Divide3/1, To Workspace2/1

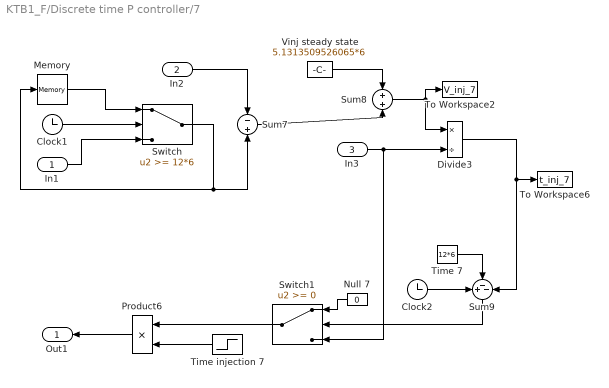
== system KTB1_F/Discrete time P controller/7 ==
  In1 : Inport
  In2 : Inport  Port=2
  In3 : Inport  Port=3
  Clock1 : Clock
  Clock2 : Clock
  Divide3 : Product  Inputs=*/
  Memory : Memory
  Null 7 : Constant  Value=0
  Product6 : Product
  Sum7 : Sum  Inputs=-+
  Sum8 : Sum
  Sum9 : Sum  Inputs=+--
  Switch : Switch  Threshold=12*6
  Switch1 : Switch
  Time 7 : Constant  Value=12*6
  Time injection 7 : Step  Time=12*6  SampleTime=0
  To Workspace2 : ToWorkspace  VariableName=V_inj_7  SaveFormat=Timeseries  SampleTime=-1
  To Workspace6 : ToWorkspace  VariableName=t_inj_7  SaveFormat=Timeseries  SampleTime=-1
  Vinj steady state : Constant  Value=5.1313509526065*6
  Out1 : Outport  VectorParamsAs1DForOutWhenUnconnected=off
  wires:
  In1/1 -> Switch/3
  Time injection 7/1 -> Product6/2
  Switch/1 -> Memory/1, Sum7/2
  Time 7/1 -> Sum9/2
  Switch1/1 -> Product6/1
  Clock1/1 -> Switch/2
  Memory/1 -> Switch/1
  Null 7/1 -> Switch1/1
  Divide3/1 -> Sum9/3, To Workspace6/1
  Clock2/1 -> Sum9/1
  In2/1 -> Sum7/1
  Vinj steady state/1 -> Sum8/1
  In3/1 -> Switch1/3, Divide3/2
  Sum9/1 -> Switch1/2
  Sum7/1 -> Sum8/2
  Product6/1 -> Out1/1
  Sum8/1 -> Divide3/1, To Workspace2/1

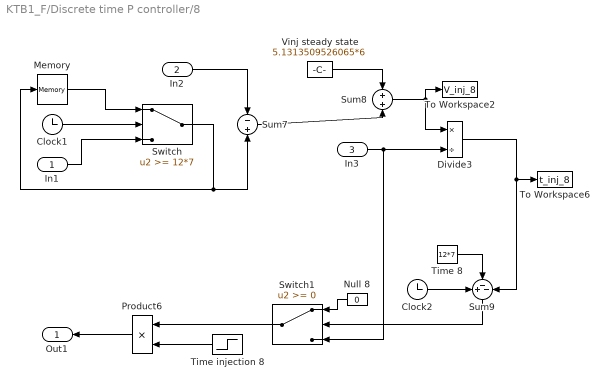
== system KTB1_F/Discrete time P controller/8 ==
  In1 : Inport
  In2 : Inport  Port=2
  In3 : Inport  Port=3
  Clock1 : Clock
  Clock2 : Clock
  Divide3 : Product  Inputs=*/
  Memory : Memory
  Null 8 : Constant  Value=0
  Product6 : Product
  Sum7 : Sum  Inputs=-+
  Sum8 : Sum
  Sum9 : Sum  Inputs=+--
  Switch : Switch  Threshold=12*7
  Switch1 : Switch
  Time 8 : Constant  Value=12*7
  Time injection 8 : Step  Time=12*7  SampleTime=0
  To Workspace2 : ToWorkspace  VariableName=V_inj_8  SaveFormat=Timeseries  SampleTime=-1
  To Workspace6 : ToWorkspace  VariableName=t_inj_8  SaveFormat=Timeseries  SampleTime=-1
  Vinj steady state : Constant  Value=5.1313509526065*6
  Out1 : Outport  VectorParamsAs1DForOutWhenUnconnected=off
  wires:
  In1/1 -> Switch/3
  Time injection 8/1 -> Product6/2
  Switch/1 -> Memory/1, Sum7/2
  Time 8/1 -> Sum9/2
  Switch1/1 -> Product6/1
  Clock1/1 -> Switch/2
  Memory/1 -> Switch/1
  Null 8/1 -> Switch1/1
  Divide3/1 -> Sum9/3, To Workspace6/1
  Clock2/1 -> Sum9/1
  In2/1 -> Sum7/1
  Vinj steady state/1 -> Sum8/1
  In3/1 -> Switch1/3, Divide3/2
  Sum9/1 -> Switch1/2
  Sum7/1 -> Sum8/2
  Product6/1 -> Out1/1
  Sum8/1 -> Divide3/1, To Workspace2/1

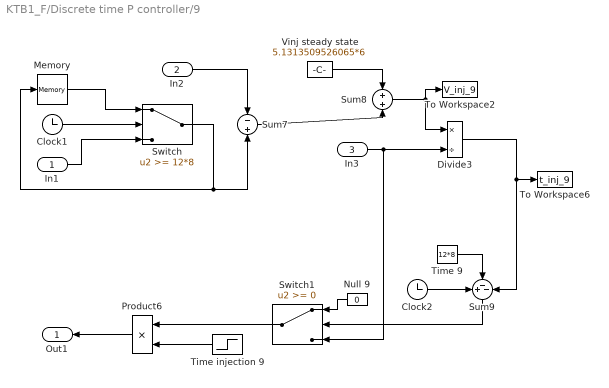
== system KTB1_F/Discrete time P controller/9 ==
  In1 : Inport
  In2 : Inport  Port=2
  In3 : Inport  Port=3
  Clock1 : Clock
  Clock2 : Clock
  Divide3 : Product  Inputs=*/
  Memory : Memory
  Null 9 : Constant  Value=0
  Product6 : Product
  Sum7 : Sum  Inputs=-+
  Sum8 : Sum
  Sum9 : Sum  Inputs=+--
  Switch : Switch  Threshold=12*8
  Switch1 : Switch
  Time 9 : Constant  Value=12*8
  Time injection 9 : Step  Time=12*8  SampleTime=0
  To Workspace2 : ToWorkspace  VariableName=V_inj_9  SaveFormat=Timeseries  SampleTime=-1
  To Workspace6 : ToWorkspace  VariableName=t_inj_9  SaveFormat=Timeseries  SampleTime=-1
  Vinj steady state : Constant  Value=5.1313509526065*6
  Out1 : Outport  VectorParamsAs1DForOutWhenUnconnected=off
  wires:
  In1/1 -> Switch/3
  Time injection 9/1 -> Product6/2
  Switch/1 -> Memory/1, Sum7/2
  Time 9/1 -> Sum9/2
  Switch1/1 -> Product6/1
  Clock1/1 -> Switch/2
  Memory/1 -> Switch/1
  Null 9/1 -> Switch1/1
  Divide3/1 -> Sum9/3, To Workspace6/1
  Clock2/1 -> Sum9/1
  In2/1 -> Sum7/1
  Vinj steady state/1 -> Sum8/1
  In3/1 -> Switch1/3, Divide3/2
  Sum9/1 -> Switch1/2
  Sum7/1 -> Sum8/2
  Product6/1 -> Out1/1
  Sum8/1 -> Divide3/1, To Workspace2/1

== matlab function KTB1_F/M-101 ==
  data: y output; u input
function y  = MX(u) 

% inputs
Q_R = u(1);
Q_M = u(2);
C_LAC_M = u(3);
C_N_M = u(4);
C_X_S = u(5);
C_LAC_S = u(6);
C_N_S = u(7);
C_MEV_S = u(8);

%C_LAC_M=10;
%C_N_M=2;

beta=1.9;

%remember C_LAC_R=C_LAC_S C_N_R=C_N_S

y=zeros(5,1);
y(1) = C_X_S*beta*Q_R/(Q_M+Q_R); %C_X_F
y(2) = (C_LAC_M*Q_M+C_LAC_S*Q_R)/(Q_M+Q_R); %C_LAC_F
y(3) = (C_N_M*Q_M+C_N_S*Q_R)/(Q_M+Q_R); %C_N_F
y(4) = C_MEV_S*Q_R/(Q_M+Q_R); %C_MEV_F
y(5) = (Q_M+Q_R); % Q_F

== matlab function KTB1_F/C-101 ==
  data: u input size=6; y output
 function y  = CF1(u)
% X=0.99; %separation factor
%Q4=QP1; volumetric capacity of the centrifuge

%inputs
C_X_T = u(1);
C_LAC_T = u(2);
C_N_T = u(3);
C_MEV_T = u(4);
Q_T = u(5);
X = u(6);

y=zeros(5,1);

y(1)=(1-X)*C_X_T;
y(2)=C_LAC_T;
y(3)=C_N_T;
y(4)=C_MEV_T;
y(5)= Q_T;

== matlab function KTB1_F/Purge ==
  data: u input size=7; y output
function y = PU(u)

% inputs
C_X_S = u(1);
C_LAC_S = u(2);
C_N_S = u(3);
C_MEV_S = u(4);
Q_M=u(5);
Q_C=u(6);
Q_P=u(7);

%F_purge=0.13;
%R=0.8;
% Q1=1.6; %l/h
%QC=1.8;
% F_purge*Q_C
%Q_P=Q_C-0.8*Q_1;

y=zeros(2,1);
y(1) = (Q_C-Q_P)/Q_M; % RR
y(2) = (Q_C-Q_P); % Q_R

== matlab function KTB1_F/C-102 ==
  data: u input size=6; y output
 function y  = CF2(u)
% X=0.99; %separation factor
%Q4=QP1; volumetric capacity of the centrifuge

%inputs
X = u(1); %separation factor
C_X_T = u(2);
C_LAC_T = u(3);
C_N_T = u(4);
C_MEV_T = u(5);
Q_T = u(6);


y=zeros(5,1);

y(1)=(1-X)*C_X_T;
y(2)=C_LAC_T;
y(3)=C_N_T;
y(4)=C_MEV_T;
y(5)= Q_T;

== matlab function KTB1_F/VSP-101 ==
  data: u input size=2; y output size=2
function y  = VSP(u)

%input
%time=u(1);
Q=u(1);
n=u(2);

dim=2;

y=zeros(dim,1);

% output

y(1)=Q;
y(2)=(-0.085*Q^2 - 0.0000329*Q*n + 0.0000155555555555556*n^2)/10.2024665317458;

% -0.085x^(2)-0.0000329*2900x+0.0000155555555555556*2900

%10.199773339984

end

== matlab function KTB1_F/NF-101 ==
  data: u input size=5; y output size=9
function y  = NF(u)
%% parameters for nanofiltration 
% a DOW NF90 nanofiltration membrane has been chosen. This type of membrane
% has been used in pharmaceutical applications for API filtrations (title
% reference: Removal of antibiotics from a model wastewater by RO/NF membranes)
%A=0.398443840087261; %membrane surface area [m^2] 
A=0.3984033;
Jw=57.90; %permeate flowrate at 8 bar pressure [l/m^2/h]
Res=Jw/8; %[l/m^2/h/bar]
% [LAC N MEV-H]


%input
C_LAC_4=u(1);
C_N_4=u(2);
C_MEV_4=u(3);
Q_IN=u(4);
P=u(5);


tlim=1; %h
dim=9;

y=zeros(dim,1);

%rejection factors based on molecular weights of similar compounds
if P<=8
    Rej=[0.9; 0.79; 0.00002*P^4 - 0.0018*P^3 + 0.0145*P^2 + 0.0849*P + 0.22248];
else
    Rej=[0.9; 0.79; 0.00002*8^4 - 0.0018*8^3 + 0.0145*8^2 + 0.0849*8 + 0.22248];
end
%Rej=[0.9; 0.79; 0.99];
% y=zeros(4,1);
% tlim=500;

%% output
%y=[Q_P2,Q_R,C_LAC_R,C_N_R,C_MEV_R,C_LAC_P2,C_N_P2,C_MEV_P2]
% if time>=0 && time<tlim
    y(1)=A*Res*P;%permeate volumetric flowrate [l/h];(ref: Continuous purification of
    %active pharmaceutical ingredients using multistage organic solvent nanofiltration membrane cascade)
    y(2)=Q_IN-y(1); %balance on centrifugation+filtration
    y(3)=(Q_IN*C_LAC_4)/(y(2)+y(1)*(1-Rej(1)));%species balance--retentate stream
    y(4)=(Q_IN*C_N_4)/(y(2)+y(1)*(1-Rej(2)));%species balance--retentate stream
    y(5)=(Q_IN*C_MEV_4)/(y(2)+y(1)*(1-Rej(3)));%species balance--retentate stream
    y(6)=y(3)*(1-Rej(1));%LAC
    y(7)=y(4)*(1-Rej(2));%N
    y(8)=y(5)*(1-Rej(3));%MEV
    y(9)=Rej(3);
%else
%    for i=1:dim
%        y(i)=0;
%    end
%end
end

== matlab function KTB1_F/HC-101 ==
  data: u input; y output
function y  = HC(u)

%inputs
Q_S=u(1);
Q_C=u(2);
C_X_S=u(3);
C_LAC_S=u(4);
C_N_S=u(5);
C_MEV_S=u(6);
% Q_R=u(7); % Serve soltanto per Fpurge, eliminabile

%parameters
%R=0.8;
beta=1.6;
%F_purge=0.13;

y=zeros(5,1);

y(1) = (C_X_S*Q_S-beta*C_X_S*Q_C)/(Q_S-Q_C); % C_X
y(2) = C_LAC_S;
y(3) = C_N_S;
y(4) = C_MEV_S;
%y(5) = 1-Q_R/Q_C;
y(5) = Q_S-Q_C;

== matlab function KTB1_F/Controller settings ==
  data: u input size=1; y output size=4
function y  = CN(u)

%inputs
err=u(1);

y=zeros(4,1);
y(1) = -2411.68044009728/310 -30*err; % P
y(2) = y(1)/599.84*1.7; % I
y(3) = -721.322122263916; % D
y(4) = 0.41482994666475; % N
